simulink model "masa_resorte_amortiguador"  (R2024a)
settings: Solver=VariableStepAuto  StartTime=0.0  StopTime=10.0  RelTol=1e-3
model workspace (MAT data in the model file):
  b = 0.8
  k1 = 1.5
  k2 = 2
  m1 = 2
  m2 = 1

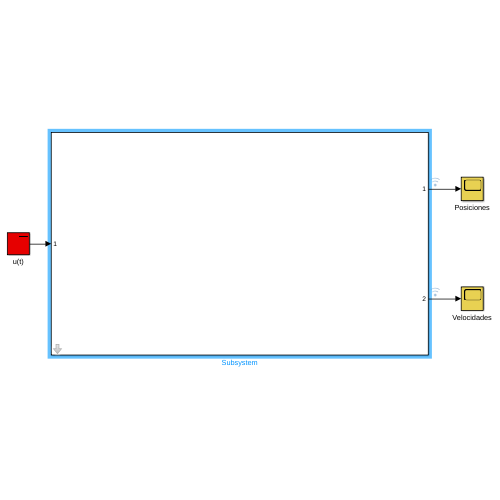
[thumbnail: Simulink's stored preview of the top-level diagram]
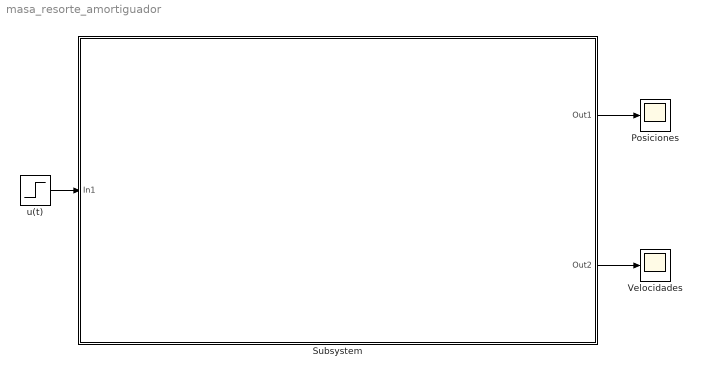
== system masa_resorte_amortiguador ==
  Posiciones : Scope
  Subsystem : Subsystem  mask{m1=2, m2=1, k1=1.5, k2=2, b=0.8}
      mask prompts: m1 "Masa 1"; m2 "Masa 2"; k1 "Const. Elastica 1"; k2 "Const. Elastica 2"; b "Const. Amortiguacion"
  Velocidades : Scope
  u(t) : Step  After=3  SampleTime=0
  wires:
  u(t)/1 -> Subsystem/1(In1)
  Subsystem/1(Out1) -> Posiciones/1
  Subsystem/2(Out2) -> Velocidades/1

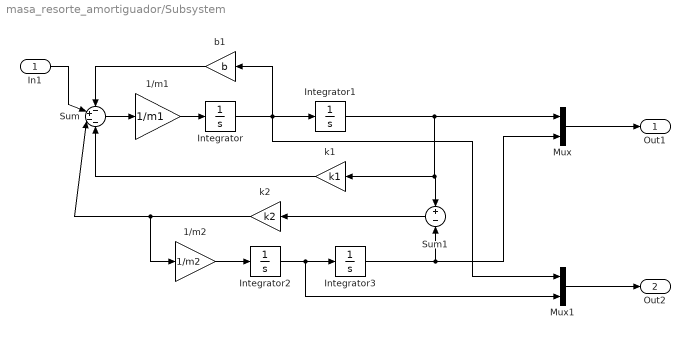
== system masa_resorte_amortiguador/Subsystem ==
  In1 : Inport
  1/m1 : Gain  Gain=1/m1
  1/m2 : Gain  Gain=1/m2
  Integrator{,1..3} (4 alike) : Integrator
  Mux : Mux  Inputs=2
  Mux1 : Mux  Inputs=2
  Sum : Sum  Inputs=-+--
  Sum1 : Sum  Inputs=+|-
  b1 : Gain  Gain=b
  k1 : Gain  Gain=k1
  k2 : Gain  Gain=k2
  Out1 : Outport
  Out2 : Outport  Port=2
  wires:
  Sum/1 -> 1/m1/1
  Mux1/1 -> Out2/1
  Integrator2/1 -> Mux1/2, Integrator3/1
  k2/1 -> Sum/3, 1/m2/1
  k1/1 -> Sum/4
  In1/1 -> Sum/2
  Integrator3/1 -> Sum1/2, Mux/2
  Integrator1/1 -> Mux/1, Sum1/1, k1/1
  Integrator/1 -> Mux1/1, b1/1, Integrator1/1
  Sum1/1 -> k2/1
  b1/1 -> Sum/1
  1/m1/1 -> Integrator/1
  1/m2/1 -> Integrator2/1
  Mux/1 -> Out1/1
